simulink model "rlKinovaBallBalance_last"  (R2024a)
settings: Solver=ode15s  StartTime=0.0  StopTime=200  RelTol=1e-3  AbsTol=1e-3
values from neighbouring files (symbols this model uses):
  max_torque = 0.75    [kinova_params.m]
  R1_q0 = 0    [kinova_params.m]
  R4_q0 = deg2rad(135)    [kinova_params.m]
  R5_q0 = 0    [kinova_params.m]
  U0 = [shoulder_torque_0 elbow_torque_0 wrist_torque_0 hand_torque_0]    [kinova_params.m]
undefined symbols (not defined in the file or in its folder): ball, Control, L1, L2, L3, LS1, LS3, plate, R1, R2, R3, Rover, rover_path, RS1, RS3, X, Y, Z
libraries: sm_lib x256, nesl_utility x104, fl_lib x85, nesl_utility_internal x30, sdl_lib x20, ee_lib x10, mars_rover_lib x6, simulink x3, slpidlib x2, batteryecm_lib x2, robotalgslib x1, rllib x1
(part 4 of 11)

== system rlKinovaBallBalance_last/Kinova Ball Balance/Rover/Chassis DOF ==
  Mux : Mux  Inputs=3
  Mux1 : Mux  Inputs=2
  Mux2 : Mux  Inputs=3
  Mux3 : Mux  Inputs=3
  PS-Simulink Converter{,1..5,7} (7 alike) : nesl_utility/PS-Simulink Converter  PhysicalDomain=network_engine_domain  SubClassName=ps_output  LeftPortType=input  RightPortType=output  PseudoPeriodic=off  Frequencies=[]  VectorFormat=1-D array  Unit=inherit  AffineConversion=off
  Rover Six Dof : sm_lib/Joints/6-DOF Joint  JointMode=Normal  CompositeWrenchDir=FollowerOnBase  CompositeWrenchFrame=BaseFrame  SenseConstraintForce=off  SenseConstraintTorque=off  SenseTotalForce=off  SenseTotalTorque=off  PxPositionTargetSpecify=on  PxPositionTargetPriority=High  PxPositionTargetValue=rover_path.x(1)  PxPositionTargetValueUnits=m  PxVelocityTargetSpecify=off  PxVelocityTargetPriority=High  PxVelocityTargetValue=0  PxVelocityTargetValueUnits=m/s  PxEquilibriumPosition=0  PxEquilibriumPositionUnits=m  PxSpringStiffness=0  PxSpringStiffnessUnits=N/m  PxDampingCoefficient=0  PxDampingCoefficientUnits=N/(m/s)  PxLowerLimitSpecify=off  PxLowerLimitBound=-1  PxLowerLimitBoundUnits=m  PxLowerLimitStiffness=1e6  PxLowerLimitStiffnessUnits=N/m  PxLowerLimitDamping=1e3  PxLowerLimitDampingUnits=N/(m/s)  PxLowerLimitTransitionRegionWidth=1e-4  PxLowerLimitTransitionRegionWidthUnits=m  PxUpperLimitSpecify=off  PxUpperLimitBound=1  PxUpperLimitBoundUnits=m  PxUpperLimitStiffness=1e6  PxUpperLimitStiffnessUnits=N/m  PxUpperLimitDamping=1e3  PxUpperLimitDampingUnits=N/(m/s)  PxUpperLimitTransitionRegionWidth=1e-4  PxUpperLimitTransitionRegionWidthUnits=m  PxTorqueActuationMode=NoTorque  PxMotionActuationMode=ComputedMotion  PxSensePosition=on  PxSenseVelocity=on  PxSenseAcceleration=off  PxSenseTorqueForce=off  PxSenseLowerLimitTorqueForce=off  PxSenseUpperLimitTorqueForce=off  PyPositionTargetSpecify=on  PyPositionTargetPriority=High  PyPositionTargetValue=rover_path.y(1)  PyPositionTargetValueUnits=m  PyVelocityTargetSpecify=off  PyVelocityTargetPriority=High  PyVelocityTargetValue=-2  PyVelocityTargetValueUnits=m/s  PyEquilibriumPosition=0  PyEquilibriumPositionUnits=m  PySpringStiffness=0  PySpringStiffnessUnits=N/m  PyDampingCoefficient=0  PyDampingCoefficientUnits=N/(m/s)  PyLowerLimitSpecify=off  PyLowerLimitBound=-1  PyLowerLimitBoundUnits=m  PyLowerLimitStiffness=1e6  PyLowerLimitStiffnessUnits=N/m  PyLowerLimitDamping=1e3  PyLowerLimitDampingUnits=N/(m/s)  PyLowerLimitTransitionRegionWidth=1e-4  PyLowerLimitTransitionRegionWidthUnits=m  PyUpperLimitSpecify=off  PyUpperLimitBound=1  PyUpperLimitBoundUnits=m  PyUpperLimitStiffness=1e6  PyUpperLimitStiffnessUnits=N/m  PyUpperLimitDamping=1e3  PyUpperLimitDampingUnits=N/(m/s)  PyUpperLimitTransitionRegionWidth=1e-4  PyUpperLimitTransitionRegionWidthUnits=m  PyTorqueActuationMode=NoTorque  PyMotionActuationMode=ComputedMotion  PySensePosition=on  PySenseVelocity=on  PySenseAcceleration=off  PySenseTorqueForce=off  PySenseLowerLimitTorqueForce=off  PySenseUpperLimitTorqueForce=off  PzPositionTargetSpecify=on  PzPositionTargetPriority=High  PzPositionTargetValue=rover_path.t0.pzOffset  PzPositionTargetValueUnits=m  PzVelocityTargetSpecify=off  PzVelocityTargetPriority=High  PzVelocityTargetValue=0  PzVelocityTargetValueUnits=m/s  PzEquilibriumPosition=0  PzEquilibriumPositionUnits=m  PzSpringStiffness=0  PzSpringStiffnessUnits=N/m  PzDampingCoefficient=0  PzDampingCoefficientUnits=N/(m/s)  PzLowerLimitSpecify=off  PzLowerLimitBound=-1  PzLowerLimitBoundUnits=m  PzLowerLimitStiffness=1e6  PzLowerLimitStiffnessUnits=N/m  PzLowerLimitDamping=1e3  PzLowerLimitDampingUnits=N/(m/s)  PzLowerLimitTransitionRegionWidth=1e-4  PzLowerLimitTransitionRegionWidthUnits=m  PzUpperLimitSpecify=off  PzUpperLimitBound=1  PzUpperLimitBoundUnits=m  PzUpperLimitStiffness=1e6  PzUpperLimitStiffnessUnits=N/m  PzUpperLimitDamping=1e3  PzUpperLimitDampingUnits=N/(m/s)  PzUpperLimitTransitionRegionWidth=1e-4  PzUpperLimitTransitionRegionWidthUnits=m  PzTorqueActuationMode=NoTorque  PzMotionActuationMode=ComputedMotion  PzSensePosition=on  PzSenseVelocity=off  PzSenseAcceleration=off  PzSenseTorqueForce=off  PzSenseLowerLimitTorqueForce=off  PzSenseUpperLimitTorqueForce=off  SphPositionTargetSpecify=on  SphPositionTargetPriority=High  SphPositionTargetRotationMethod=RotationSequence  SphPositionTargetFollAlignAxisA=+X  SphPositionTargetBaseAlignAxisA=+Y  SphPositionTargetFollAlignAxisB=+Y  SphPositionTargetBaseAlignAxisB=+Z  SphPositionTargetRotationStandardAxis=+X  SphPositionTargetRotationAngle=0.0647207  SphPositionTargetRotationAngleUnits=rad  SphPositionTargetRotationArbitraryAxis=[0.195566 -0.656945 0.728133]  SphPositionTargetRotationSequenceAxes=FollowerAxes  SphPositionTargetRotationSequence=ZYX  SphPositionTargetRotationSequenceAngles="[rover_path.t0.yaw  rover_path.t0.pitch  rover_path.t0.roll]"  SphPositionTargetRotationSequenceAnglesUnits=rad  SphPositionTargetRotationMatrix=[1 0 0; 0 1 0; 0 0 1]  SphPositionTargetQuaternion=[1 0 0 0]  SphVelocityTargetSpecify=off  SphVelocityTargetPriority=High  SphVelocityTargetValue=[0 0 45]  SphVelocityTargetValueUnits=deg/s  SphVelocityTargetInFollowerFrame=on  SphEqPosRotationMethod=None  SphEqPosFollAlignAxisA=+X  SphEqPosBaseAlignAxisA=+Y  SphEqPosFollAlignAxisB=+Y  SphEqPosBaseAlignAxisB=+Z  SphEqPosRotationStandardAxis=+Z  SphEqPosRotationAngle=0.0  SphEqPosRotationAngleUnits=deg  SphEqPosRotationArbitraryAxis=[0 0 1]  SphEqPosRotationSequenceAxes=FollowerAxes  SphEqPosRotationSequence=XYX  SphEqPosRotationSequenceAngles=[0 0 0]  SphEqPosRotationSequenceAnglesUnits=deg  SphEqPosRotationMatrix=[1 0 0; 0 1 0; 0 0 1]  SphEqPosQuaternion=[1 0 0 0]  SphSpringStiffness=0  SphSpringStiffnessUnits=m*N/deg  SphDampingCoefficient=0  SphDampingCoefficientUnits=m*s*N/deg  SphLowerLimitSpecify=off  SphLowerLimitBound=15  SphLowerLimitBoundUnits=deg  SphLowerLimitStiffness=1e4  SphLowerLimitStiffnessUnits=N*m/deg  SphLowerLimitDamping=10  SphLowerLimitDampingUnits=N*m/(deg/s)  SphLowerLimitTransitionRegionWidth=0.1  SphLowerLimitTransitionRegionWidthUnits=deg  SphUpperLimitSpecify=off  SphUpperLimitBound=45  SphUpperLimitBoundUnits=deg  SphUpperLimitStiffness=1e4  SphUpperLimitStiffnessUnits=N*m/deg  SphUpperLimitDamping=10  SphUpperLimitDampingUnits=N*m/(deg/s)  SphUpperLimitTransitionRegionWidth=0.1  SphUpperLimitTransitionRegionWidthUnits=deg  SphTorqueActuationMode=NoTorque  SphActuateTorqueX=off  SphActuateTorqueY=off  SphActuateTorqueZ=off  SphActuateTorque=off  SphActuationFrame=BaseFrame  SphSensePosition=on  SphSenseVelocityX=off  SphSenseVelocityY=off  SphSenseVelocityZ=on  SphSenseVelocity=off  SphSenseAccelerationX=off  SphSenseAccelerationY=off  SphSenseAccelerationZ=off  SphSenseAcceleration=off  SphSenseLowerLimitTorqueMag=off  SphSenseUpperLimitTorqueMag=off  SphSensingFrame=BaseFrame
  Sqrt : Sqrt
  Square : Math  Operator=square
  Square1 : Math  Operator=square
  Sum : Sum  Inputs=|++
  theta_act : MATLAB Function  TreatAsAtomicUnit=on
  F : PMIOPort  Side=Right
  B : PMIOPort  Port=2  Side=Left
  Out Bus Element : Outport  PortName=m  Element=Pose
  Out Bus Element1 : Outport  PortName=m  Element=xyz
  Out Bus Element2 : Outport  PortName=m  Element=vxy
  Out Bus Element3 : Outport  PortName=m  Element=rpy
  Out Bus Element4 : Outport  PortName=m  Element=wz
  Out Bus Element5 : Outport  PortName=m  Element=v
  wires:
  theta_act/1(z) -> Mux2/3, Mux/3
  PS-Simulink Converter/1 -> theta_act/1(u)
  Mux2/1 -> Out Bus Element3/1
  Mux1/1 -> Out Bus Element2/1
  Mux3/1 -> Out Bus Element1/1
  PS-Simulink Converter7/1 -> Mux3/3
  theta_act/2(y) -> Mux2/2
  Mux/1 -> Out Bus Element/1
  PS-Simulink Converter5/1 -> Mux3/1, Mux/1  "RoverPosX"
  PS-Simulink Converter4/1 -> Out Bus Element4/1
  theta_act/3(x) -> Mux2/1
  PS-Simulink Converter1/1 -> Mux3/2, Mux/2  "RoverPosY"
  PS-Simulink Converter2/1 -> Square/1, Mux1/1
  Square1/1 -> Sum/2
  Square/1 -> Sum/1
  PS-Simulink Converter3/1 -> Square1/1, Mux1/2
  Sum/1 -> Sqrt/1
  Sqrt/1 -> Out Bus Element5/1
  connections:
  F/RConn1 -- Rover Six Dof/RConn1
  B/RConn1 -- Rover Six Dof/LConn1
  PS-Simulink Converter/LConn1 -- Rover Six Dof/RConn7
  PS-Simulink Converter4/LConn1 -- Rover Six Dof/RConn8
  PS-Simulink Converter5/LConn1 -- Rover Six Dof/RConn2
  PS-Simulink Converter1/LConn1 -- Rover Six Dof/RConn4
  PS-Simulink Converter7/LConn1 -- Rover Six Dof/RConn6
  PS-Simulink Converter2/LConn1 -- Rover Six Dof/RConn3
  PS-Simulink Converter3/LConn1 -- Rover Six Dof/RConn5

== system rlKinovaBallBalance_last/Kinova Ball Balance/Rover/Path ==
  Points : sm_lib/Curves and Surfaces/Point Cloud  CoordinatesMatrix=[rover_path.x rover_path.y rover_path.z]  CoordinatesMatrixUnits=m  GraphicType=MarkerCloud  GraphicSphereRadius=0.05*3  GraphicSphereRadiusUnits=m  GraphicVisPropType=SimpleVisualProperties  GraphicDiffuseColor=[0 0 1]  GraphicOpacity=1  GraphicSpecularColor=[0.5 0.5 0.5 1.0]  GraphicAmbientColor=[0.15 0.15 0.15 1.0]  GraphicEmissiveColor=[0.0 0.0 0.0 1.0]  GraphicShininess=75
  Rigid Transform : sm_lib/Frames and Transforms/Rigid Transform  RotationMethod=None  FollAlignAxisA=+X  BaseAlignAxisA=+Y  FollAlignAxisB=+Y  BaseAlignAxisB=+Z  RotationStandardAxis=+Z  RotationAngle=0.0  RotationAngleUnits=deg  RotationArbitraryAxis=[0 0 1]  RotationSequenceAxes=FollowerAxes  RotationSequence=XYX  RotationSequenceAngles=[0 0 0]  RotationSequenceAnglesUnits=deg  RotationMatrix=[1 0 0; 0 1 0; 0 0 1]  Quaternion=[1 0 0 0]  TranslationMethod=StandardAxis  TranslationCartesianOffset=[0 0 0]  TranslationCartesianOffsetUnits=m  TranslationStandardAxis=+Z  TranslationStandardOffset=rover_path.Offset_vis_z  TranslationStandardOffsetUnits=m  TranslationROffset=0  TranslationROffsetUnits=m  TranslationThetaOffset=0  TranslationThetaOffsetUnits=deg  TranslationZOffset=0  TranslationZOffsetUnits=m
  Spline : sm_lib/Curves and Surfaces/Spline  Commented=on  DataPoints=u  DataPointsUnits=m  EndConditionType=Natural  GraphicType=FromGeometry  MarkerShape=Sphere  MarkerSize=10  GraphicVisPropType=SimpleVisualProperties  GraphicDiffuseColor=[0.1294 0.5333 0.8196]  GraphicOpacity=1  GraphicSpecularColor=[0.5 0.5 0.5 1.0]  GraphicAmbientColor=[0.15 0.15 0.15 1.0]  GraphicEmissiveColor=[0.0 0.0 0.0 1.0]  GraphicShininess=75
  R : PMIOPort  Side=Left
  connections:
  Rigid Transform/RConn1 -- Spline/LConn1 -- Points/LConn1
  R/RConn1 -- Rigid Transform/LConn1

== system rlKinovaBallBalance_last/Kinova Ball Balance/Rover/Terrain ==
  note: Uncomment for additional terrain visualization options.
  Contact : Subsystem  mask{contact_k=Rover.Wheel_Surface.Contact.k, contact_d=Rover.Wheel_Surface.Contact.d, contact_tw=Rover.Wheel_Surface.Contact.trans_depth, friction_mus=Rover.Wheel_Surface.Friction.mu_static, friction_mud=Rover.Wheel_Surface.Friction.mu_dynamic, friction_vcrit=Rover.Wheel_Surface.Friction.vel_crit}
      mask prompts: contact_k "Stiffness (N/m)"; contact_d "Damping (N/(m/s))"; contact_tw "Transition Region Width (m)"; friction_mus "Coefficient of Static Friction"; friction_mud "Coefficient of Dynamic Friction"; friction_vcrit "Critical Velocity (m/s)"
      mask DialogControl cont_contact Prompt: Contact Parameters
      mask DialogControl cont_friction Prompt: Contact Friction
  Terrain Geometry : sm_lib/Body Elements/File Solid  Commented=on  ExtGeomFileName=mars_terrain.stl  UnitType=Custom  ExtGeomFileUnits=m  StepReaderType=HEX  ExportConvexHullGeometry=off  InertiaType=CalculateFromGeometry  BasedOnType=Mass  Density=1000  DensityUnits=kg/m^3  Mass=1  MassUnits=kg  CenterOfMass=[0 0 0]  CenterOfMassUnits=m  MomentsOfInertia=[1 1 1]  MomentsOfInertiaUnits=kg*m^2  ProductsOfInertia=[0 0 0]  ProductsOfInertiaUnits=kg*m^2  GraphicType=FromGeometry  MarkerShape=Sphere  MarkerSize=10  GraphicVisPropType=SimpleVisualProperties  GraphicDiffuseColor=[1.0 0.6 0.6]  GraphicOpacity=1.0  GraphicSpecularColor=[0.5 0.5 0.5 1.0]  GraphicAmbientColor=[0.15 0.15 0.15 1.0]  GraphicEmissiveColor=[0.0 0.0 0.0 1.0]  GraphicShininess=75  DoExposeReferenceFrame=on  SerializedFrames=<Frames/>
  Terrain Point Cloud : sm_lib/Curves and Surfaces/Point Cloud  Commented=on  CoordinatesMatrix=mars_terrain_grid.ptcloud  CoordinatesMatrixUnits=m  GraphicType=MarkerCloud  GraphicSphereRadius=0.03  GraphicSphereRadiusUnits=m  GraphicVisPropType=SimpleVisualProperties  GraphicDiffuseColor=[0 1 0]  GraphicOpacity=1.0  GraphicSpecularColor=[0.5 0.5 0.5 1.0]  GraphicAmbientColor=[0.15 0.15 0.15 1.0]  GraphicEmissiveColor=[0.0 0.0 0.0 1.0]  GraphicShininess=75
  Terrain Grid Surface : sm_lib/Curves and Surfaces/Grid Surface  XGridVector=mars_terrain_grid.xg  XGridVectorUnits=m  YGridVector=mars_terrain_grid.yg  YGridVectorUnits=m  ZHeights=mars_terrain_grid.z_heights  ZHeightsUnits=m  GraphicType=FromGeometry  GraphicVisPropType=SimpleVisualProperties  GraphicDiffuseColor=[187 109 63]/255*1.3  GraphicOpacity=1  GraphicSpecularColor=[0.5 0.5 0.5 1.0]  GraphicAmbientColor=[0.15 0.15 0.15 1.0]  GraphicEmissiveColor=[0.0 0.0 0.0 1.0]  GraphicShininess=75
  W : PMIOPort  Side=Right
  G : PMIOPort  Port=2  Side=Right
  connections:
  W/RConn1 -- Terrain Point Cloud/LConn1 -- Terrain Geometry/RConn1 -- Terrain Grid Surface/LConn1
  Contact/RConn1 -- G/RConn1
  Contact/RConn2 -- Terrain Grid Surface/RConn1

== system rlKinovaBallBalance_last/Kinova Ball Balance/7 DOF Manipulator/Bracelet_Link/Bracelet Link ==
  FileSolid : Subsystem  VariantControl=Choice_1
  Inertia : Subsystem  VariantControl=Choice
  R : PMIOPort  Side=Right

== system rlKinovaBallBalance_last/Kinova Ball Balance/7 DOF Manipulator/ForeArm_Link/ForeArm Link ==
  FileSolid : Subsystem  VariantControl=Choice_1
  Inertia : Subsystem  VariantControl=Choice
  R : PMIOPort  Side=Right

== system rlKinovaBallBalance_last/Kinova Ball Balance/7 DOF Manipulator/HalfArm1_Link/HalfArm1 Link ==
  FileSolid : Subsystem  VariantControl=Choice_1
  Inertia : Subsystem  VariantControl=Choice
  R : PMIOPort  Side=Right

== system rlKinovaBallBalance_last/Kinova Ball Balance/7 DOF Manipulator/HalfArm2_Link/HalfArm2 Link ==
  FileSolid : Subsystem  VariantControl=Choice_1
  Inertia : Subsystem  VariantControl=Choice
  R : PMIOPort  Side=Right

== system rlKinovaBallBalance_last/Kinova Ball Balance/7 DOF Manipulator/Shoulder_Link/Shoulder Link ==
  FileSolid : Subsystem  VariantControl=Choice_1
  Inertia : Subsystem  VariantControl=Choice
  R : PMIOPort  Side=Right

== system rlKinovaBallBalance_last/Kinova Ball Balance/7 DOF Manipulator/Wrist1_Link/Wrist1 Link ==
  FileSolid : Subsystem  VariantControl=Choice_1
  Inertia : Subsystem  VariantControl=Choice
  R : PMIOPort  Side=Right

== system rlKinovaBallBalance_last/Kinova Ball Balance/7 DOF Manipulator/Wrist2_Link/Wrist2 Link ==
  FileSolid : Subsystem  VariantControl=Choice_1
  Inertia : Subsystem  VariantControl=Choice
  R : PMIOPort  Side=Right

== system rlKinovaBallBalance_last/Kinova Ball Balance/7 DOF Manipulator/base_link/Base Link ==
  FileSolid : Subsystem  VariantControl=Choice_1
  Inertia : Subsystem  VariantControl=Choice
  R : PMIOPort  Side=Right

== system rlKinovaBallBalance_last/Kinova Ball Balance/Control/Chassis Control/Ackerman Steer Angle ==
  note: ROC: Radius of Curvature
      | A3: Axle 3
      | L3: Rear Left Wheel
      | R3: Rear Right Wheel
  AtGoal : Inport
  Delta : Inport  Port=2
  Ackerman Steering Angle Formulation : MATLAB Function  TreatAsAtomicUnit=on
  Clock1 : Clock
  Constant : Constant  Value=Rover.Chassis.Length/2
  Constant3 : Constant  Value=0
  Constant4 : Constant  Value=Rover.Chassis.Width
  Gain3 : Gain  Gain=-1
  Gain4 : Gain  Gain=-1
  Hold Steer at Goal : Subsystem  TreatAsAtomicUnit=on
  Mux : Mux
  NOT : Logic  Operator=NOT  IconShape=distinctive  AllPortsSameDT=off  OutDataTypeStr=boolean
  Saturation{1..4} (4 alike) : Saturate  UpperLimit=60  LowerLimit=-60
  Scope : Scope  NumInputPorts=3
  Switch2 : Switch  Criteria=u2 > Threshold  Threshold=1  SaturateOnIntegerOverflow=off  InputSameDT=off
  AckSteerAngs : Outport
  A3 ROC : Outport  Port=2
  L3ROC : Outport  Port=3
  R3ROC : Outport  Port=4
  wires:
  Delta/1 -> Switch2/1
  Ackerman Steering Angle Formulation/2(qSteerR3) -> Scope/3, Saturation3/1, Gain4/1
  Ackerman Steering Angle Formulation/5(R_R) -> R3ROC/1
  Saturation4/1 -> Mux/4  "R1"
  Saturation1/1 -> Mux/2  "L1"
  Hold Steer at Goal/1(d_h) -> Scope/1, Ackerman Steering Angle Formulation/1(delta)
  Ackerman Steering Angle Formulation/1(qSteerL3) -> Scope/2, Saturation2/1, Gain3/1
  Constant/1 -> Ackerman Steering Angle Formulation/2(L)
  Saturation3/1 -> Mux/3  "R3"
  Mux/1 -> AckSteerAngs/1
  Clock1/1 -> Switch2/2
  Switch2/1 -> Hold Steer at Goal/1(d)
  Gain4/1 -> Saturation4/1
  Saturation2/1 -> Mux/1  "L3"
  Constant4/1 -> Ackerman Steering Angle Formulation/3(d)
  Gain3/1 -> Saturation1/1
  Ackerman Steering Angle Formulation/4(L_R) -> L3ROC/1
  Ackerman Steering Angle Formulation/3(R) -> A3 ROC/1
  Constant3/1 -> Switch2/3
  AtGoal/1 -> NOT/1
  NOT/1 -> Hold Steer at Goal/Enable

== system rlKinovaBallBalance_last/Kinova Ball Balance/Control/Chassis Control/Steering Controller ==
  Meas : Inport
  qSteerWhl : Inport  Port=2
  RoverAtGoal : Inport  Port=3
  Add : Sum  Inputs=+-
  Bus to Vec : Subsystem
  Check Difference : Subsystem
  Constant : Constant  Value=[Kp Ki]
  Constant1 : Constant  Value=[10 1 ]
  Constant2 : Constant  Value=Kd
  Constant3 : Constant  Value=N
  Demux : Demux  Outputs=2
  Demux1 : Demux
  Filter qMeas : Subsystem  mask(First-order lag supporting vector signals){b=[1 1 1 1]*Ts_Measq, x_initial=[0 0 0 0]}
      mask prompts: b "Filter time constant"; x_initial "Initial output"
      mask help: Models a lag of the form 1/(b*s+1) where s is the Laplace operator.
  Filter qTarget : Subsystem  mask(First-order lag supporting vector signals){b=[1 1 1 1]*Ts_Targetq, x_initial=[0 0 0 0]}
      mask prompts: b "Filter time constant"; x_initial "Initial output"
      mask help: Models a lag of the form 1/(b*s+1) where s is the Laplace operator.
  PID Controller : slpidlib/PID Controller  Controller=PID  Form=Parallel  TimeDomain=Continuous-time  UseExternalTs=off  SampleTime=-1  IntegratorMethod=Forward Euler  FilterMethod=Forward Euler  ControllerParametersSource=external  P=1  I=0  UseKiTs=off  D=0  UseExternalDerivativeSource=off  N=10  UseFilter=on  TunerSelectOption=Transfer Function Based (PID Tuner App)  InitialConditionSource=internal  InitialConditionForIntegrator=0  InitialConditionForFilter=0  DifferentiatorICPrevScaledInput=0  ExternalReset=none  TrackingMode=off  Kt=1  LimitOutput=on  SatLimitsSource=internal  UpperSaturationLimit=trq_max_pos  LowerSaturationLimit=trq_max_neg  LinearizeAsGain=on  AntiWindupMode=none  Kb=1  LimitIntegrator=off  UpperIntegratorSaturationLimit=inf  LowerIntegratorSaturationLimit=-inf  POutMin=[]  POutMax=[]  IOutMin=[]  IOutMax=[]  DOutMin=[]  DOutMax=[]  NOutMin=[]  NOutMax=[]  SumOutMin=[]  SumOutMax=[]  SaturationOutMin=[]  SaturationOutMax=[]  PParamMin=[]  PParamMax=[]  IParamMin=[]  IParamMax=[]  DParamMin=[]  DParamMax=[]  NParamMin=[]  NParamMax=[]  KbParamMin=[]  KbParamMax=[]  KtParamMin=[]  KtParamMax=[]  KbOutMin=[]  KbOutMax=[]  KtOutMin=[]  KtOutMax=[]  IntegratorOutMin=[]  IntegratorOutMax=[]  FilterOutMin=[]  FilterOutMax=[]  SumI1OutMin=[]  SumI1OutMax=[]  SumI2OutMin=[]  SumI2OutMax=[]  SumI3OutMin=[]  SumI3OutMax=[]  SumI4OutMin=[]  SumI4OutMax=[]  SumDOutMin=[]  SumDOutMax=[]  DifferentiatorOutMin=[]  DifferentiatorOutMax=[]  FilterDiffOutCoefMin=[]  FilterDiffOutCoefMax=[]  ReciprocalOutMin=[]  ReciprocalOutMax=[]  SumDenOutMin=[]  SumDenOutMax=[]  SumNumOutMin=[]  SumNumOutMax=[]  DivideOutMin=[]  DivideOutMax=[]  UdiffTsProdOutMin=[]  UdiffTsProdOutMax=[]  NTsProdOutMin=[]  NTsProdOutMax=[]  UintegralTsProdOutMin=[]  UintegralTsProdOutMax=[]  UngainTsProdOutMin=[]  UngainTsProdOutMax=[]  ClampingZeroOutDataTypeStr=Inherit: Inherit via back propagation  ClampingZeroOutMin=[]  ClampingZeroOutMax=[]  FilterDenConstantOutDataTypeStr=Inherit: Inherit via back propagation  FilterDenConstantOutMin=[]  FilterDenConstantOutMax=[]  PCopyOutDataTypeStr=Inherit: Inherit via back propagation  PCopyOutMin=[]  PCopyOutMax=[]  NCopyOutDataTypeStr=Inherit: Inherit via back propagation  NCopyOutMin=[]  NCopyOutMax=[]  IntegratorContinuousStateAttributes=''  IntegratorStateMustResolveToSignalObject=off  IntegratorRTWStateStorageClass=Auto  FilterContinuousStateAttributes=''  FilterStateMustResolveToSignalObject=off  FilterRTWStateStorageClass=Auto  ParallelPVariant=ExternalParameters  IdealPVariant=Disabled  IVariant=ExternalParameters  DVariant=ExternalParameters  IntegratorVariant=Continuous  SatVariant=Enabled  AWVariant=Passthrough  PCopyVariant=Disabled  TRVariant=Disabled  FdbkBlocksVariant=Forward  IdealPFdbkVariant=Disabled  SatFdbkVariant=Disabled  DerivativeFilterVariant=ContFilter  NVariant=ExternalParameters  NCopyVariant=Disabled  FilterICVariant=InternalICsFilter  IntegratorICVariant=InternalICs  ExternalResetVariant=Disabled  TRSumVariant=Passthrough  SumFdbkVariant=Disabled  SumVariant=Sum_PID  TsampFilterVariant=InternalTs  TsampNgainVariant=Passthrough  TsampIntegralVariant=Disabled_SignalSpec  ExternalSaturationOutDataTypeStr=Inherit: Same as second input  DerivativeSourceVariant=ErrorSignal
  Scope : Scope  NumInputPorts=4
  Scope1 : Scope  NumInputPorts=4
  Switch : Switch  Criteria=u2 > Threshold  SaturateOnIntegerOverflow=off  InputSameDT=off
  trq : Outport
  wires:
  PID Controller/1 -> trq/1
  qSteerWhl/1 -> Filter qTarget/1(In)
  Add/1 -> PID Controller/1, Demux1/1
  RoverAtGoal/1 -> Switch/2
  Constant1/1 -> Switch/1
  Demux/1 -> PID Controller/2
  Demux/2 -> PID Controller/3
  Constant/1 -> Switch/3
  Switch/1 -> Demux/1
  Meas/1 -> Bus to Vec/1(B)
  Bus to Vec/1(V) -> Filter qMeas/1(In)
  Check Difference/1(L3) -> Scope/1
  Check Difference/2(L1) -> Scope/2
  Check Difference/3(R3) -> Scope/3
  Check Difference/4(R1) -> Scope/4
  Constant2/1 -> PID Controller/4
  Filter qMeas/1(Out) -> Check Difference/2(meas), Add/2
  Filter qTarget/1(Out) -> Add/1, Check Difference/1(tgt)
  Demux1/1 -> Scope1/1
  Demux1/2 -> Scope1/2
  Demux1/3 -> Scope1/3
  Demux1/4 -> Scope1/4
  Constant3/1 -> PID Controller/5

== system rlKinovaBallBalance_last/Kinova Ball Balance/Control/Chassis Control/Target Dir To Bicycle Steer Angle ==
  TargetDir : Inport
  Bicycle length : Constant  Value=L
  Constant : Constant  Value=2
  Divide : Product  Inputs=*/
  Lookahead distance : Constant  Value=ld
  Product : Product
  Product1 : Product
  Rad2Deg : MATLAB Function  TreatAsAtomicUnit=on
  Scope : Scope  NumInputPorts=4
  Sine Wave : Sin  TimeSource=Use external signal  SampleTime=0
  Trigonometric Function : Trigonometry  Operator=atan
  qSteer : Outport
  wires:
  Sine Wave/1 -> Product1/2, Scope/2
  Bicycle length/1 -> Product/2
  Constant/1 -> Product/1
  Product1/1 -> Divide/1
  Product/1 -> Product1/1
  Divide/1 -> Trigonometric Function/1
  Trigonometric Function/1 -> Scope/3, Rad2Deg/1(u)
  TargetDir/1 -> Scope/1, Sine Wave/1
  Lookahead distance/1 -> Divide/2
  Rad2Deg/1(y) -> Scope/4, qSteer/1

== system rlKinovaBallBalance_last/Kinova Ball Balance/Control/Chassis Control/Target Direction and Speed ==
  vRover : Inport
  Pose : Inport  Port=2
  WP : Inport  Port=3
  AND : Logic  IconShape=distinctive  AllPortsSameDT=off  OutDataTypeStr=boolean
  Check Distance To Goal : Subsystem
  Check for Stop : simulink/Logic and Bit Operations/Compare To Constant  relop=<=  const=0.05  OutDataTypeStr=boolean
  Clock3 : Clock
  Constant10 : Constant  Value=Control.Drive.StartTime
  Constant11 : Constant  Value=Control.Drive.TargetAccel
  Constant7 : Constant  Value=[rover_path.x(end) rover_path.y(end)]
  Demux : Demux  Outputs=3
  Pure Pursuit Control : robotalgslib/Pure Pursuit  DesiredLinearVelocityPort=off  DesiredLinearVelocity=Control.Drive.TargetSpeed  MaxAngularVelocity=0.01  LookaheadDistancePort=off  LookaheadDistance=0.75  TargetDirPort=on  SimulateUsing=Code generation
  Scope : Scope  NumInputPorts=2
  Scope1 : Scope  NumInputPorts=3
  Terminator : Terminator
  Transfer Fcn : TransferFcn  Denominator=[0.1 1]
  Transfer Fcn1 : TransferFcn  Denominator=[0.5 1]
  Trapezoidal Vel Profile : MATLAB Function  TreatAsAtomicUnit=on
  hold : Subsystem
  StopAtGoal : Outport
  vTarget : Outport  Port=2
  AtGoal : Outport  Port=3
  TargetDir : Outport  Port=4
  wires:
  hold/1(Out1) -> Trapezoidal Vel Profile/4(deaccelStartTime)
  Pure Pursuit Control/1 -> Trapezoidal Vel Profile/5(linVel), Check Distance To Goal/3(linVel)
  Constant11/1 -> Trapezoidal Vel Profile/3(accel)
  Constant7/1 -> Check Distance To Goal/1(goal)
  Check Distance To Goal/1(atGoal) -> AtGoal/1, AND/2
  Clock3/1 -> Trapezoidal Vel Profile/1(t)
  Check for Stop/1 -> AND/1
  Pose/1 -> Demux/1, Check Distance To Goal/2(currentPose), Pure Pursuit Control/1
  Pure Pursuit Control/2 -> Terminator/1
  Constant10/1 -> Trapezoidal Vel Profile/2(startTime)
  Check Distance To Goal/2(Slow) -> hold/1(In1)
  AND/1 -> StopAtGoal/1
  WP/1 -> Pure Pursuit Control/2
  Trapezoidal Vel Profile/1(lin_Vel_out) -> Transfer Fcn/1
  Transfer Fcn/1 -> vTarget/1
  Transfer Fcn1/1 -> Scope/2, TargetDir/1
  vRover/1 -> Check for Stop/1
  Demux/1 -> Scope1/1
  Demux/2 -> Scope1/2
  Demux/3 -> Scope1/3
  Pure Pursuit Control/3 -> Scope/1, Transfer Fcn1/1

== system rlKinovaBallBalance_last/Kinova Ball Balance/Control/Chassis Control/Vec to Bus SteerTrq ==
  V : Inport
  Bus Creator : BusCreator  Inputs=4
  Demux : Demux
  B : Outport
  wires:
  Demux/3 -> Bus Creator/3  "R3"
  Bus Creator/1 -> B/1
  V/1 -> Demux/1
  Demux/4 -> Bus Creator/4  "R1"
  Demux/1 -> Bus Creator/1  "L3"
  Demux/2 -> Bus Creator/2  "L1"

== system rlKinovaBallBalance_last/Kinova Ball Balance/Control/Chassis Control/Vec to Bus qSteer ==
  V : Inport
  Bus Creator : BusCreator  Inputs=4
  Demux : Demux
  B : Outport
  wires:
  Demux/2 -> Bus Creator/2  "L1"
  Demux/4 -> Bus Creator/4  "R1"
  Demux/3 -> Bus Creator/3  "R3"
  Demux/1 -> Bus Creator/1  "L3"
  Bus Creator/1 -> B/1
  V/1 -> Demux/1

== system rlKinovaBallBalance_last/Kinova Ball Balance/Control/Chassis Control/Vec to Bus trq ==
  V : Inport
  Bus Creator : BusCreator  Inputs=6
  Demux : Demux  Outputs=6
  B : Outport
  wires:
  Demux/5 -> Bus Creator/5  "R2"
  Demux/2 -> Bus Creator/2  "L2"
  Demux/6 -> Bus Creator/6  "R3"
  Demux/1 -> Bus Creator/1  "L1"
  Demux/4 -> Bus Creator/4  "R1"
  V/1 -> Demux/1
  Bus Creator/1 -> B/1
  Demux/3 -> Bus Creator/3  "L3"

== system rlKinovaBallBalance_last/Kinova Ball Balance/Control/Chassis Control/Vec to Bus wWhl ==
  V : Inport
  Bus Creator : BusCreator  Inputs=6
  Demux : Demux  Outputs=6
  B : Outport
  wires:
  V/1 -> Demux/1
  Bus Creator/1 -> B/1
  Demux/1 -> Bus Creator/1  "L1"
  Demux/3 -> Bus Creator/3  "L3"
  Demux/4 -> Bus Creator/4  "R1"
  Demux/2 -> Bus Creator/2  "L2"
  Demux/5 -> Bus Creator/5  "R2"
  Demux/6 -> Bus Creator/6  "R3"

== system rlKinovaBallBalance_last/Kinova Ball Balance/Control/Chassis Control/Wheel Speed Controller ==
  Meas : Inport
  StopAtGoal : Inport  Port=2
  wTarget : Inport  Port=3
  Add3 : Sum  Inputs=+-
  Bus to Vec : Subsystem
  Constant : Constant  Value=[Kp,Ki]
  Constant1 : Constant  Value=[5000 100]
  Constant2 : Constant  Value=Kd
  Constant3 : Constant  Value=N
  Demux : Demux  Outputs=2
  Filter wMeas : Subsystem  mask(First-order lag supporting vector signals){b=[1 1 1 1 1 1]*Ts_Measw, x_initial=[0 0 0 0 0 0]}
      mask prompts: b "Filter time constant"; x_initial "Initial output"
      mask help: Models a lag of the form 1/(b*s+1) where s is the Laplace operator.
  Filter wTarget : Subsystem  mask(First-order lag supporting vector signals){b=[1 1 1 1 1 1]*Ts_Targetw, x_initial=[0 0 0 0 0 0]}
      mask prompts: b "Filter time constant"; x_initial "Initial output"
      mask help: Models a lag of the form 1/(b*s+1) where s is the Laplace operator.
  PID Controller : slpidlib/PID Controller  Controller=PID  Form=Parallel  TimeDomain=Continuous-time  UseExternalTs=off  SampleTime=-1  IntegratorMethod=Forward Euler  FilterMethod=Forward Euler  ControllerParametersSource=external  P=1  I=0  UseKiTs=off  D=0  UseExternalDerivativeSource=off  N=100  UseFilter=on  TunerSelectOption=Transfer Function Based (PID Tuner App)  InitialConditionSource=internal  InitialConditionForIntegrator=0  InitialConditionForFilter=0  DifferentiatorICPrevScaledInput=0  ExternalReset=none  TrackingMode=off  Kt=1  LimitOutput=off  SatLimitsSource=internal  UpperSaturationLimit=inf  LowerSaturationLimit=-inf  LinearizeAsGain=on  AntiWindupMode=none  Kb=1  LimitIntegrator=off  UpperIntegratorSaturationLimit=inf  LowerIntegratorSaturationLimit=-inf  POutMin=[]  POutMax=[]  IOutMin=[]  IOutMax=[]  DOutMin=[]  DOutMax=[]  NOutMin=[]  NOutMax=[]  SumOutMin=[]  SumOutMax=[]  SaturationOutMin=[]  SaturationOutMax=[]  PParamMin=[]  PParamMax=[]  IParamMin=[]  IParamMax=[]  DParamMin=[]  DParamMax=[]  NParamMin=[]  NParamMax=[]  KbParamMin=[]  KbParamMax=[]  KtParamMin=[]  KtParamMax=[]  KbOutMin=[]  KbOutMax=[]  KtOutMin=[]  KtOutMax=[]  IntegratorOutMin=[]  IntegratorOutMax=[]  FilterOutMin=[]  FilterOutMax=[]  SumI1OutMin=[]  SumI1OutMax=[]  SumI2OutMin=[]  SumI2OutMax=[]  SumI3OutMin=[]  SumI3OutMax=[]  SumI4OutMin=[]  SumI4OutMax=[]  SumDOutMin=[]  SumDOutMax=[]  DifferentiatorOutMin=[]  DifferentiatorOutMax=[]  FilterDiffOutCoefMin=[]  FilterDiffOutCoefMax=[]  ReciprocalOutMin=[]  ReciprocalOutMax=[]  SumDenOutMin=[]  SumDenOutMax=[]  SumNumOutMin=[]  SumNumOutMax=[]  DivideOutMin=[]  DivideOutMax=[]  UdiffTsProdOutMin=[]  UdiffTsProdOutMax=[]  NTsProdOutMin=[]  NTsProdOutMax=[]  UintegralTsProdOutMin=[]  UintegralTsProdOutMax=[]  UngainTsProdOutMin=[]  UngainTsProdOutMax=[]  ClampingZeroOutDataTypeStr=Inherit: Inherit via back propagation  ClampingZeroOutMin=[]  ClampingZeroOutMax=[]  FilterDenConstantOutDataTypeStr=Inherit: Inherit via back propagation  FilterDenConstantOutMin=[]  FilterDenConstantOutMax=[]  PCopyOutDataTypeStr=Inherit: Inherit via back propagation  PCopyOutMin=[]  PCopyOutMax=[]  NCopyOutDataTypeStr=Inherit: Inherit via back propagation  NCopyOutMin=[]  NCopyOutMax=[]  IntegratorContinuousStateAttributes=''  IntegratorStateMustResolveToSignalObject=off  IntegratorRTWStateStorageClass=Auto  FilterContinuousStateAttributes=''  FilterStateMustResolveToSignalObject=off  FilterRTWStateStorageClass=Auto  ParallelPVariant=ExternalParameters  IdealPVariant=Disabled  IVariant=ExternalParameters  DVariant=ExternalParameters  IntegratorVariant=Continuous  SatVariant=Disabled  AWVariant=Passthrough  PCopyVariant=Disabled  TRVariant=Disabled  FdbkBlocksVariant=Forward  IdealPFdbkVariant=Disabled  SatFdbkVariant=Disabled  DerivativeFilterVariant=ContFilter  NVariant=ExternalParameters  NCopyVariant=Disabled  FilterICVariant=InternalICsFilter  IntegratorICVariant=InternalICs  ExternalResetVariant=Disabled  TRSumVariant=Passthrough  SumFdbkVariant=Disabled  SumVariant=Sum_PID  TsampFilterVariant=InternalTs  TsampNgainVariant=Passthrough  TsampIntegralVariant=Disabled_SignalSpec  ExternalSaturationOutDataTypeStr=Inherit: Same as second input  DerivativeSourceVariant=ErrorSignal
  Saturation : Saturate  UpperLimit=trq_max_pos  LowerLimit=trq_max_neg
  Switch : Switch  Criteria=u2 > Threshold  SaturateOnIntegerOverflow=off  InputSameDT=off
  trq : Outport
  wires:
  Switch/1 -> Demux/1
  Constant/1 -> Switch/3
  Constant1/1 -> Switch/1
  Demux/2 -> PID Controller/3
  Demux/1 -> PID Controller/2
  StopAtGoal/1 -> Switch/2
  PID Controller/1 -> Saturation/1
  Meas/1 -> Bus to Vec/1(B)
  Add3/1 -> PID Controller/1
  Saturation/1 -> trq/1
  Bus to Vec/1(V) -> Filter wMeas/1(In)
  wTarget/1 -> Filter wTarget/1(In)
  Constant2/1 -> PID Controller/4
  Constant3/1 -> PID Controller/5
  Filter wMeas/1(Out) -> Add3/2
  Filter wTarget/1(Out) -> Add3/1

== system rlKinovaBallBalance_last/Kinova Ball Balance/Rover/Chassis/Bar L ==
  Connecting Bar L : sm_lib/Body Elements/Brick Solid  BrickDimensions=[1 20.000000607487117 1]  BrickDimensionsUnits=cm  ExportEntireGeometry=off  InertiaType=CalculateFromGeometry  BasedOnType=Density  Density=2700  DensityUnits=kg/m^3  Mass=3  MassUnits=kg  CenterOfMass=[0 0 0]  CenterOfMassUnits=m  MomentsOfInertia=[1 1 1]  MomentsOfInertiaUnits=kg*m^2  ProductsOfInertia=[0 0 0]  ProductsOfInertiaUnits=kg*m^2  GraphicType=FromGeometry  MarkerShape=Sphere  MarkerSize=10  GraphicVisPropType=SimpleVisualProperties  GraphicDiffuseColor=[0.5 0.5 0.5]  GraphicOpacity=1.0  GraphicSpecularColor=[0.5 0.5 0.5 1.0]  GraphicAmbientColor=[0.15 0.15 0.15 1.0]  GraphicEmissiveColor=[0.0 0.0 0.0 1.0]  GraphicShininess=75  DoExposeReferenceFrame=off  SerializedFrames=<Frames><Frame><Id>Frame1</Id><Value><Name>F1</Name><Origin><Source>GeometricFeature</Source><FeatureName>-y surface</FeatureName></Origin><PrimaryAxis><DefinedDirection>+Z</DefinedDirection><Source>ReferenceFrame</Source><SourceDirection>+Z</SourceDirection><FeatureName></FeatureName></PrimaryAxis><SecondaryAxis><DefinedDirection>+X</DefinedDirection><Source>ReferenceFrame</Source><SourceDirection>+X</SourceDirection><FeatureName></FeatureName></SecondaryAxis></Value></Frame><Frame><Id>Frame2</Id><Value><Name>F2</Name><Origin><Source>GeometricFeature</Source><FeatureName>+y surface</FeatureName></Origin><PrimaryAxis><DefinedDirection>+Z</DefinedDirection><Source>ReferenceFrame</Source><SourceDirection>+X</SourceDirection><FeatureName></FeatureName></PrimaryAxis><SecondaryAxis><DefinedDirection>+X</DefinedDirection><Source>ReferenceFrame</Source><SourceDirection>-Y</SourceDirection><FeatureName></FeatureName></SecondaryAxis></Value></Frame></Frames>
  Rigid Transform2 : sm_lib/Frames and Transforms/Rigid Transform  RotationMethod=StandardAxis  FollAlignAxisA=+X  BaseAlignAxisA=+Y  FollAlignAxisB=+Y  BaseAlignAxisB=+Z  RotationStandardAxis=+X  RotationAngle=90  RotationAngleUnits=deg  RotationArbitraryAxis=[0 0 1]  RotationSequenceAxes=FollowerAxes  RotationSequence=XYX  RotationSequenceAngles=[0 0 0]  RotationSequenceAnglesUnits=deg  RotationMatrix=[1 0 0; 0 1 0; 0 0 1]  Quaternion=[1 0 0 0]  TranslationMethod=None  TranslationCartesianOffset=[0 0 0]  TranslationCartesianOffsetUnits=m  TranslationStandardAxis=+Z  TranslationStandardOffset=0  TranslationStandardOffsetUnits=m  TranslationROffset=0  TranslationROffsetUnits=m  TranslationThetaOffset=0  TranslationThetaOffsetUnits=deg  TranslationZOffset=0  TranslationZOffsetUnits=m
  Rigid Transform4 : sm_lib/Frames and Transforms/Rigid Transform  RotationMethod=None  FollAlignAxisA=+X  BaseAlignAxisA=+Y  FollAlignAxisB=+Y  BaseAlignAxisB=+Z  RotationStandardAxis=+X  RotationAngle=180  RotationAngleUnits=deg  RotationArbitraryAxis=[0 0 1]  RotationSequenceAxes=FollowerAxes  RotationSequence=XYX  RotationSequenceAngles=[0 0 0]  RotationSequenceAnglesUnits=deg  RotationMatrix=[1 0 0; 0 1 0; 0 0 1]  Quaternion=[1 0 0 0]  TranslationMethod=None  TranslationCartesianOffset=[0 0 0]  TranslationCartesianOffsetUnits=m  TranslationStandardAxis=+Z  TranslationStandardOffset=0  TranslationStandardOffsetUnits=m  TranslationROffset=0  TranslationROffsetUnits=m  TranslationThetaOffset=0  TranslationThetaOffsetUnits=deg  TranslationZOffset=0  TranslationZOffsetUnits=m
  B : PMIOPort  Side=Left
  F : PMIOPort  Port=2  Side=Right
  connections:
  Rigid Transform4/LConn1 -- Rigid Transform2/LConn1
  Connecting Bar L/LConn1 -- Rigid Transform4/RConn1
  Rigid Transform2/RConn1 -- B/RConn1
  Connecting Bar L/RConn1 -- F/RConn1

== system rlKinovaBallBalance_last/Kinova Ball Balance/Rover/Chassis/Bar R ==
  Connecting Bar R : sm_lib/Body Elements/Brick Solid  BrickDimensions=[1 20.000000607487117 1]  BrickDimensionsUnits=cm  ExportEntireGeometry=off  InertiaType=CalculateFromGeometry  BasedOnType=Density  Density=2700  DensityUnits=kg/m^3  Mass=3  MassUnits=kg  CenterOfMass=[0 0 0]  CenterOfMassUnits=m  MomentsOfInertia=[1 1 1]  MomentsOfInertiaUnits=kg*m^2  ProductsOfInertia=[0 0 0]  ProductsOfInertiaUnits=kg*m^2  GraphicType=FromGeometry  MarkerShape=Sphere  MarkerSize=10  GraphicVisPropType=SimpleVisualProperties  GraphicDiffuseColor=[0.5 0.5 0.5]  GraphicOpacity=1.0  GraphicSpecularColor=[0.5 0.5 0.5 1.0]  GraphicAmbientColor=[0.15 0.15 0.15 1.0]  GraphicEmissiveColor=[0.0 0.0 0.0 1.0]  GraphicShininess=75  DoExposeReferenceFrame=off  SerializedFrames=<Frames><Frame><Id>Frame1</Id><Value><Name>F1</Name><Origin><Source>GeometricFeature</Source><FeatureName>-y surface</FeatureName></Origin><PrimaryAxis><DefinedDirection>+Z</DefinedDirection><Source>ReferenceFrame</Source><SourceDirection>+Z</SourceDirection><FeatureName></FeatureName></PrimaryAxis><SecondaryAxis><DefinedDirection>+X</DefinedDirection><Source>ReferenceFrame</Source><SourceDirection>+X</SourceDirection><FeatureName></FeatureName></SecondaryAxis></Value></Frame><Frame><Id>Frame2</Id><Value><Name>F2</Name><Origin><Source>GeometricFeature</Source><FeatureName>+y surface</FeatureName></Origin><PrimaryAxis><DefinedDirection>+Z</DefinedDirection><Source>ReferenceFrame</Source><SourceDirection>+X</SourceDirection><FeatureName></FeatureName></PrimaryAxis><SecondaryAxis><DefinedDirection>+X</DefinedDirection><Source>ReferenceFrame</Source><SourceDirection>+Y</SourceDirection><FeatureName></FeatureName></SecondaryAxis></Value></Frame></Frames>
  Rigid Transform2 : sm_lib/Frames and Transforms/Rigid Transform  RotationMethod=StandardAxis  FollAlignAxisA=+X  BaseAlignAxisA=+Y  FollAlignAxisB=+Y  BaseAlignAxisB=+Z  RotationStandardAxis=+X  RotationAngle=90  RotationAngleUnits=deg  RotationArbitraryAxis=[0 0 1]  RotationSequenceAxes=FollowerAxes  RotationSequence=XYX  RotationSequenceAngles=[0 0 0]  RotationSequenceAnglesUnits=deg  RotationMatrix=[1 0 0; 0 1 0; 0 0 1]  Quaternion=[1 0 0 0]  TranslationMethod=None  TranslationCartesianOffset=[0 0 0]  TranslationCartesianOffsetUnits=m  TranslationStandardAxis=+Z  TranslationStandardOffset=0  TranslationStandardOffsetUnits=m  TranslationROffset=0  TranslationROffsetUnits=m  TranslationThetaOffset=0  TranslationThetaOffsetUnits=deg  TranslationZOffset=0  TranslationZOffsetUnits=m
  Rigid Transform3 : sm_lib/Frames and Transforms/Rigid Transform  RotationMethod=StandardAxis  FollAlignAxisA=+X  BaseAlignAxisA=+Y  FollAlignAxisB=+Y  BaseAlignAxisB=+Z  RotationStandardAxis=+X  RotationAngle=180  RotationAngleUnits=deg  RotationArbitraryAxis=[0 0 1]  RotationSequenceAxes=FollowerAxes  RotationSequence=XYX  RotationSequenceAngles=[0 0 0]  RotationSequenceAnglesUnits=deg  RotationMatrix=[1 0 0; 0 1 0; 0 0 1]  Quaternion=[1 0 0 0]  TranslationMethod=None  TranslationCartesianOffset=[0 0 0]  TranslationCartesianOffsetUnits=m  TranslationStandardAxis=+Z  TranslationStandardOffset=0  TranslationStandardOffsetUnits=m  TranslationROffset=0  TranslationROffsetUnits=m  TranslationThetaOffset=0  TranslationThetaOffsetUnits=deg  TranslationZOffset=0  TranslationZOffsetUnits=m
  B : PMIOPort  Side=Left
  F : PMIOPort  Port=2  Side=Right
  connections:
  Connecting Bar R/LConn1 -- Rigid Transform3/RConn1
  B/RConn1 -- Rigid Transform2/RConn1
  F/RConn1 -- Connecting Bar R/RConn1
  Rigid Transform2/LConn1 -- Rigid Transform3/LConn1

== system rlKinovaBallBalance_last/Kinova Ball Balance/Rover/Chassis/Bogie L ==
  Bogie : sm_lib/Body Elements/File Solid  ExtGeomFileName=rover_chassis_bogie_left.stl  UnitType=Custom  ExtGeomFileUnits=cm  StepReaderType=HEX  ExportConvexHullGeometry=off  InertiaType=CalculateFromGeometry  BasedOnType=Density  Density=1000  DensityUnits=kg/m^3  Mass=0  MassUnits=kg  CenterOfMass=[0 0 0]  CenterOfMassUnits=m  MomentsOfInertia=[1 1 1]*0  MomentsOfInertiaUnits=kg*m^2  ProductsOfInertia=[0 0 0]  ProductsOfInertiaUnits=kg*m^2  GraphicType=FromGeometry  MarkerShape=Sphere  MarkerSize=10  GraphicVisPropType=AdvancedVisualProperties  GraphicDiffuseColor=[0.2 0.2 0.3]  GraphicOpacity=1.0  GraphicSpecularColor=[1 1 1 1.0]  GraphicAmbientColor=[0.15 0.15 0.15 1.0]  GraphicEmissiveColor=[0.0 0.0 0.0 1.0]  GraphicShininess=90  DoExposeReferenceFrame=on  SerializedFrames=<Frames/>
  Reference Frame : sm_lib/Frames and Transforms/Reference Frame
  Rigid Transform1 : sm_lib/Frames and Transforms/Rigid Transform  RotationMethod=StandardAxis  FollAlignAxisA=+X  BaseAlignAxisA=+Y  FollAlignAxisB=+Y  BaseAlignAxisB=+Z  RotationStandardAxis=+Z  RotationAngle=90  RotationAngleUnits=deg  RotationArbitraryAxis=[0 0 1]  RotationSequenceAxes=FollowerAxes  RotationSequence=XYX  RotationSequenceAngles=[0 0 0]  RotationSequenceAnglesUnits=deg  RotationMatrix=[1 0 0; 0 1 0; 0 0 1]  Quaternion=[1 0 0 0]  TranslationMethod=None  TranslationCartesianOffset=[0 0 0]  TranslationCartesianOffsetUnits=m  TranslationStandardAxis=+Z  TranslationStandardOffset=0  TranslationStandardOffsetUnits=m  TranslationROffset=0  TranslationROffsetUnits=m  TranslationThetaOffset=0  TranslationThetaOffsetUnits=deg  TranslationZOffset=0  TranslationZOffsetUnits=m
  Rigid Transform2 : sm_lib/Frames and Transforms/Rigid Transform  RotationMethod=RotationMatrix  FollAlignAxisA=+X  BaseAlignAxisA=+Y  FollAlignAxisB=+Y  BaseAlignAxisB=+Z  RotationStandardAxis=+Z  RotationAngle=0.0  RotationAngleUnits=deg  RotationArbitraryAxis=[0 0 1]  RotationSequenceAxes=FollowerAxes  RotationSequence=XYX  RotationSequenceAngles=[0 0 0]  RotationSequenceAnglesUnits=deg  RotationMatrix=Rover.BogieL.PSJ_R  Quaternion=[1 0 0 0]  TranslationMethod=Cartesian  TranslationCartesianOffset=Rover.BogieL.PSJ_T  TranslationCartesianOffsetUnits=m  TranslationStandardAxis=+Z  TranslationStandardOffset=0  TranslationStandardOffsetUnits=m  TranslationROffset=0  TranslationROffsetUnits=m  TranslationThetaOffset=0  TranslationThetaOffsetUnits=deg  TranslationZOffset=0  TranslationZOffsetUnits=m
  Rigid Transform3 : sm_lib/Frames and Transforms/Rigid Transform  RotationMethod=None  FollAlignAxisA=+X  BaseAlignAxisA=+Y  FollAlignAxisB=+Y  BaseAlignAxisB=+Z  RotationStandardAxis=+Z  RotationAngle=0.0  RotationAngleUnits=deg  RotationArbitraryAxis=[0 0 1]  RotationSequenceAxes=FollowerAxes  RotationSequence=XYX  RotationSequenceAngles=[0 0 0]  RotationSequenceAnglesUnits=deg  RotationMatrix=Rover.BogieL.SLB_R  Quaternion=[1 0 0 0]  TranslationMethod=Cartesian  TranslationCartesianOffset=Rover.BogieL.SLB_T  TranslationCartesianOffsetUnits=m  TranslationStandardAxis=+Z  TranslationStandardOffset=0  TranslationStandardOffsetUnits=m  TranslationROffset=0  TranslationROffsetUnits=m  TranslationThetaOffset=0  TranslationThetaOffsetUnits=deg  TranslationZOffset=0  TranslationZOffsetUnits=m
  Rigid Transform4 : sm_lib/Frames and Transforms/Rigid Transform  RotationMethod=RotationMatrix  FollAlignAxisA=+X  BaseAlignAxisA=+Y  FollAlignAxisB=+Y  BaseAlignAxisB=+Z  RotationStandardAxis=+Z  RotationAngle=0.0  RotationAngleUnits=deg  RotationArbitraryAxis=[0 0 1]  RotationSequenceAxes=FollowerAxes  RotationSequence=XYX  RotationSequenceAngles=[0 0 0]  RotationSequenceAnglesUnits=deg  RotationMatrix=Rover.BogieL.SLM_R  Quaternion=[1 0 0 0]  TranslationMethod=Cartesian  TranslationCartesianOffset=Rover.BogieL.SLM_T  TranslationCartesianOffsetUnits=m  TranslationStandardAxis=+Z  TranslationStandardOffset=0  TranslationStandardOffsetUnits=m  TranslationROffset=0  TranslationROffsetUnits=m  TranslationThetaOffset=0  TranslationThetaOffsetUnits=deg  TranslationZOffset=0  TranslationZOffsetUnits=m
  D : PMIOPort  Side=Right
  S : PMIOPort  Port=2  Side=Right
  R : PMIOPort  Port=3  Side=Left
  connections:
  Bogie/RConn1 -- Rigid Transform4/LConn1 -- Rigid Transform2/LConn1 -- Rigid Transform3/LConn1 -- Reference Frame/RConn1
  R/RConn1 -- Rigid Transform2/RConn1
  D/RConn1 -- Rigid Transform4/RConn1
  Rigid Transform1/LConn1 -- Rigid Transform3/RConn1
  S/RConn1 -- Rigid Transform1/RConn1

== system rlKinovaBallBalance_last/Kinova Ball Balance/Rover/Chassis/Bogie R ==
  Bogie : sm_lib/Body Elements/File Solid  ExtGeomFileName=rover_chassis_bogie_right.stl  UnitType=Custom  ExtGeomFileUnits=cm  StepReaderType=HEX  ExportConvexHullGeometry=off  InertiaType=CalculateFromGeometry  BasedOnType=Density  Density=1000  DensityUnits=kg/m^3  Mass=0  MassUnits=kg  CenterOfMass=[0 0 0]  CenterOfMassUnits=m  MomentsOfInertia=[1 1 1]*0  MomentsOfInertiaUnits=kg*m^2  ProductsOfInertia=[0 0 0]  ProductsOfInertiaUnits=kg*m^2  GraphicType=FromGeometry  MarkerShape=Sphere  MarkerSize=10  GraphicVisPropType=AdvancedVisualProperties  GraphicDiffuseColor=[0.2 0.2 0.3]  GraphicOpacity=1.0  GraphicSpecularColor=[1 1 1 1.0]  GraphicAmbientColor=[0.15 0.15 0.15 1.0]  GraphicEmissiveColor=[0.0 0.0 0.0 1.0]  GraphicShininess=90  DoExposeReferenceFrame=on  SerializedFrames=<Frames/>
  Reference Frame : sm_lib/Frames and Transforms/Reference Frame
  Rigid Transform1 : sm_lib/Frames and Transforms/Rigid Transform  RotationMethod=RotationMatrix  FollAlignAxisA=+X  BaseAlignAxisA=+Y  FollAlignAxisB=+Y  BaseAlignAxisB=+Z  RotationStandardAxis=+Z  RotationAngle=0.0  RotationAngleUnits=deg  RotationArbitraryAxis=[0 0 1]  RotationSequenceAxes=FollowerAxes  RotationSequence=XYX  RotationSequenceAngles=[0 0 0]  RotationSequenceAnglesUnits=deg  RotationMatrix=Rover.BogieR.SRM_R  Quaternion=[1 0 0 0]  TranslationMethod=Cartesian  TranslationCartesianOffset=Rover.BogieR.SRM_T  TranslationCartesianOffsetUnits=m  TranslationStandardAxis=+Z  TranslationStandardOffset=0  TranslationStandardOffsetUnits=m  TranslationROffset=0  TranslationROffsetUnits=m  TranslationThetaOffset=0  TranslationThetaOffsetUnits=deg  TranslationZOffset=0  TranslationZOffsetUnits=m
  Rigid Transform2 : sm_lib/Frames and Transforms/Rigid Transform  RotationMethod=RotationMatrix  FollAlignAxisA=+X  BaseAlignAxisA=+Y  FollAlignAxisB=+Y  BaseAlignAxisB=+Z  RotationStandardAxis=+Z  RotationAngle=0.0  RotationAngleUnits=deg  RotationArbitraryAxis=[0 0 1]  RotationSequenceAxes=FollowerAxes  RotationSequence=XYX  RotationSequenceAngles=[0 0 0]  RotationSequenceAnglesUnits=deg  RotationMatrix=Rover.BogieR.PSJ_R  Quaternion=[1 0 0 0]  TranslationMethod=Cartesian  TranslationCartesianOffset=Rover.BogieR.PSJ_T  TranslationCartesianOffsetUnits=m  TranslationStandardAxis=+Z  TranslationStandardOffset=0  TranslationStandardOffsetUnits=m  TranslationROffset=0  TranslationROffsetUnits=m  TranslationThetaOffset=0  TranslationThetaOffsetUnits=deg  TranslationZOffset=0  TranslationZOffsetUnits=m
  Rigid Transform3 : sm_lib/Frames and Transforms/Rigid Transform  RotationMethod=StandardAxis  FollAlignAxisA=+X  BaseAlignAxisA=+Y  FollAlignAxisB=+Y  BaseAlignAxisB=+Z  RotationStandardAxis=+Z  RotationAngle=-90  RotationAngleUnits=deg  RotationArbitraryAxis=[0 0 1]  RotationSequenceAxes=FollowerAxes  RotationSequence=XYX  RotationSequenceAngles=[0 0 0]  RotationSequenceAnglesUnits=deg  RotationMatrix=[1 0 0; 0 1 0; 0 0 1]  Quaternion=[1 0 0 0]  TranslationMethod=None  TranslationCartesianOffset=[0 0 0]  TranslationCartesianOffsetUnits=m  TranslationStandardAxis=+Z  TranslationStandardOffset=0  TranslationStandardOffsetUnits=m  TranslationROffset=0  TranslationROffsetUnits=m  TranslationThetaOffset=0  TranslationThetaOffsetUnits=deg  TranslationZOffset=0  TranslationZOffsetUnits=m
  Rigid Transform4 : sm_lib/Frames and Transforms/Rigid Transform  RotationMethod=RotationMatrix  FollAlignAxisA=+X  BaseAlignAxisA=+Y  FollAlignAxisB=+Y  BaseAlignAxisB=+Z  RotationStandardAxis=+Z  RotationAngle=0.0  RotationAngleUnits=deg  RotationArbitraryAxis=[0 0 1]  RotationSequenceAxes=FollowerAxes  RotationSequence=XYX  RotationSequenceAngles=[0 0 0]  RotationSequenceAnglesUnits=deg  RotationMatrix=Rover.BogieR.SRB_R  Quaternion=[1 0 0 0]  TranslationMethod=Cartesian  TranslationCartesianOffset=Rover.BogieR.SRB_T  TranslationCartesianOffsetUnits=m  TranslationStandardAxis=+Z  TranslationStandardOffset=0  TranslationStandardOffsetUnits=m  TranslationROffset=0  TranslationROffsetUnits=m  TranslationThetaOffset=0  TranslationThetaOffsetUnits=deg  TranslationZOffset=0  TranslationZOffsetUnits=m
  Transform Right Side : sm_lib/Frames and Transforms/Rigid Transform  RotationMethod=StandardAxis  FollAlignAxisA=+X  BaseAlignAxisA=+Y  FollAlignAxisB=+Y  BaseAlignAxisB=+Z  RotationStandardAxis=+Y  RotationAngle=180  RotationAngleUnits=deg  RotationArbitraryAxis=[0 0 1]  RotationSequenceAxes=FollowerAxes  RotationSequence=XYX  RotationSequenceAngles=[0 0 0]  RotationSequenceAnglesUnits=deg  RotationMatrix=[1 0 0; 0 1 0; 0 0 1]  Quaternion=[1 0 0 0]  TranslationMethod=None  TranslationCartesianOffset=[0 0 0]  TranslationCartesianOffsetUnits=m  TranslationStandardAxis=+Z  TranslationStandardOffset=0  TranslationStandardOffsetUnits=m  TranslationROffset=0  TranslationROffsetUnits=m  TranslationThetaOffset=0  TranslationThetaOffsetUnits=deg  TranslationZOffset=0  TranslationZOffsetUnits=m
  D : PMIOPort  Side=Left
  S : PMIOPort  Port=2  Side=Left
  R : PMIOPort  Port=3  Side=Right
  connections:
  S/RConn1 -- Rigid Transform3/RConn1
  Rigid Transform2/RConn1 -- R/RConn1
  Rigid Transform1/RConn1 -- Transform Right Side/RConn1
  Rigid Transform3/LConn1 -- Rigid Transform4/RConn1
  Bogie/RConn1 -- Rigid Transform1/LConn1 -- Rigid Transform4/LConn1 -- Rigid Transform2/LConn1 -- Reference Frame/RConn1
  Transform Right Side/LConn1 -- D/RConn1
